simulink model "Trajectory_tracking_4th_order"  (R2024a)
settings: Solver=VariableStepAuto  StartTime=0.0  StopTime=tf  RelTol=1e-3
InitFcn:
  | %% Define the points of the curve
  | x=xp;
  | y=yp;
  | 
  | % Number of points
  | n = length(x);
  | 
  | % Initialize the arclength array
  | s = zeros(1, n);
  | 
  | %% Compute the incremental distances and the cumulative sum
  | for i = 2:n
  |     ds = sqrt((x(i) - x(i-1))^2 + (y(i) - y(i-1))^2);
  |     s(i) = s(i-1) + ds;
  | end
  | 
  | s= s/max(s);
  | 
  | [s, unique_indices] = unique(s, 'stable');
  | x = x(unique_indices);
  | y = y(unique_indices);
  | 
  | n = length(x);
  | 
  | %% Compute derivatives with respect to s
  | dx_ds = gradient(x, s);
  | dy_ds = gradient(y, s);
  | 
  | % Compute second derivatives with respect to s
  | d2x_ds2 = gradient(dx_ds, s);
  | d2y_ds2 = gradient(dy_ds, s);
  | 
  | % Compute third derivatives with respect to s
  | d3x_ds3 = gradient(d2x_ds2, s);
  | d3y_ds3 = gradient(d2y_ds2, s);
  | 
  | curvature = sqrt(d2x_ds2.^2+d2y_ds2.^2);
  | 
  | % % Dati Robot
  | %CGTF=0.325;
  | %CGTR=0.325;
  | Ts = 1/n;
  | 
  | 
  | %% Calcolo path
  | x_s= x;
  | y_s= y;
  | 
  | x_s_prime = dx_ds;
  | y_s_prime = dy_ds;
  | 
  | x_s_second = d2x_ds2;
  | y_s_second = d2y_ds2;
  | 
  | x_s_third = d3x_ds3;
  | y_s_third = d3y_ds3;
  | 
  | v_tilde = sqrt(x_s_prime.^2 + y_s_prime.^2);
  | 
  | theta_s = atan2(y_s_prime./v_tilde,x_s_prime./v_tilde);
  | theta_s_prime = (y_s_second.*x_s_prime-x_s_second.*y_s_prime)./(v_tilde.^2);
  | 
  | phi_s = atan(l*(y_s_second.*x_s_prime-x_s_second.*y_s_prime)./(v_tilde.^3));
  | 
  | w_tilde = (l*v_tilde.*((y_s_third.*x_s_prime-x_s_third.*y_s_prime)-3*(y_s_second.*x_s_prime-x_s_second.*y_s_prime).*(x_s_prime.*x_s_second+y_s_prime.*y_s_second)))./((v_tilde.^6)+(l^2)*(y_s_second.*x_s_prime-x_s_second.*y_s_prime).^2);
  | 
  | %% Time law
  | check=0;
  | t0 = 0;
  | %tf = 1;
  | K=1;
  | while (~check)
  | 
  |     a0 = s(:,1);
  |     a1 = 0;
  |     a2 = 3/(tf^2)*(s(:,n)-s(:,1));
  |     a3 = -2/(tf^3)*(s(:,n)-s(:,1));
  | 
  |     % % Define the boundary conditions for s(t)
  |     % t0 = 0; % initial time
  |     % t_end = tf; % end time
  |     % s0 = s(:,1); % initial arc length
  |     % s_end = s(:,n); % end arc length
  |     % v0 = 0; % initial velocity
  |     % v_end = 0; % end velocity
  |     % a0 = 0; % initial acceleration
  |     % a_end = 0; % end acceleration
  |     %
  |     % % Set up the system of equations for quintic polynomial
  |     % A = [
  |     %     1, t0, t0^2, t0^3, t0^4, t0^5;
  |     %     1, t_end, t_end^2, t_end^3, t_end^4, t_end^5;
  |     %     0, 1, 2*t0, 3*t0^2, 4*t0^3, 5*t0^4;
  |     %     0, 1, 2*t_end, 3*t_end^2, 4*t_end^3, 5*t_end^4;
  |     %     0, 0, 2, 6*t0, 12*t0^2, 20*t0^3;
  |     %     0, 0, 2, 6*t_end, 12*t_end^2, 20*t_end^3
  |     % ];
  |     %
  |     % b = [s0; s_end; v0; v_end; a0; a_end];
  |     %
  |     % % Solve for the coefficients
  |     % coefficients = A\b;
  |     %
  |     % % Extract the coefficients
  |     % a0 = coefficients(1);
  |     % a1 = coefficients(2);
  |     % a2 = coefficients(3);
  |     % a3 = coefficients(4);
  |     % a4 = coefficients(5);
  |     % a5 = coefficients(6);
  | 
  |     % Define the quintic polynomial function s(t)
  |     % s_t = @(t) a0 + a1*t + a2*t^2 + a3*t^3 + a4*t^4 + a5*t^5;
  |     s_t = @(t) a3*t^3 + a2*t^2 + a1*t + a0;
  | 
  |     % Create x(t) and y(t)
  |     x_t = @(t) interp1(s, x_s, s_t(t),'spline','extrap');
  |     y_t = @(t) interp1(s, y_s, s_t(t),'spline','extrap');
  | 
  |     t_values = linspace(0, tf, n);
  | 
  |     x_values = arrayfun(@(t) x_t(t),t_values);
  |     y_values = arrayfun(@(t) y_t(t),t_values);
  | 
  |     s_t_dot = 3*a3*t_values.^2 + 2*a2*t_values + a1;
  |     % s_t_dot = a1 + 2*a2*t_values + 3*a3*t_values.^2 + 4*a4*t_values.^3 + 5*a5*t_values.^4;
  | 
  |     x_t_dot = x_s_prime.*s_t_dot;
  |     y_t_dot = y_s_prime.*s_t_dot;
  | 
  |     v_t = v_tilde.*s_t_dot;
  | 
  |     w_t = w_tilde.*s_t_dot;
  | 
  |     theta_t = @(t) interp1(s, theta_s, s_t(t),'spline','extrap');
  |     theta_values = arrayfun(@(t) theta_t(t),t_values);
  | 
  |     theta_t_dot = theta_s_prime.*s_t_dot;
  | 
  |     phi_t = @(t) interp1(s, phi_s, s_t(t),'spline','extrap');
  |     phi_values = arrayfun(@(t) phi_t(t),t_values);
  | 
  |     theta_t_dot_lim = tan(phi_lim)/l*vlim;
  | 
  |     v_max = max(abs(v_t));
  |     w_max = max(abs(w_t));
  |     theta_max = max(abs(theta_t_dot));
  |     phi_max = max(abs(phi_values));
  | 
  |     check = 1;
  | 
  |     if ((v_max>vlim || w_max>wlim || theta_max>theta_t_dot_lim)) %&& phi_max<phi_lim )
  |         Kmax = [v_max/vlim w_max/wlim theta_max/theta_t_dot_lim ];
  |         K = max(Kmax);
  |         tf = tf*K;
  |         check=0;
  |     end
  | 
  | end
  | 
  | 
  | v_t_reference = timeseries(v_t,t_values);
  | w_t_reference = timeseries(w_t,t_values);
  | theta_t_reference = timeseries(theta_values,t_values);
  | theta_t_dot_reference = timeseries(theta_t_dot,t_values);
  | phi_t_reference = timeseries(phi_values,t_values);
  | 
  | x_t_reference = timeseries(x_values,t_values);
  | y_t_reference = timeseries(y_values,t_values);
  | x_dot_t_reference = timeseries(x_t_dot,t_values);
  | y_dot_t_reference = timeseries(y_t_dot,t_values);
values from neighbouring files (symbols this model uses):
  b = 5    [main.m]
  k1 = 30    [main.m]
  k2 = 3    [main.m]
undefined symbols (not defined in the file or in its folder): l, phi_lim, vlim, wlim
settings Model: Creator=arsen  LastModifiedBy=arsen

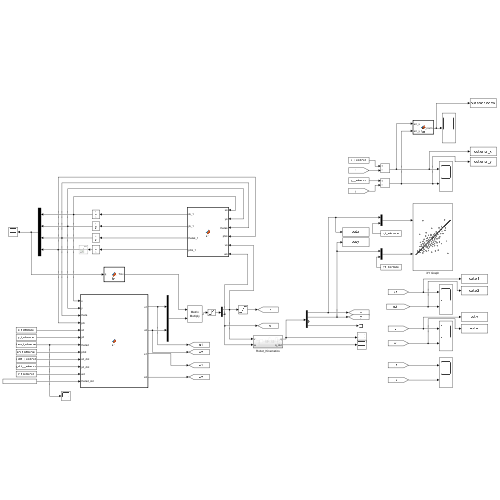
[thumbnail: Simulink's stored preview of the top-level diagram]
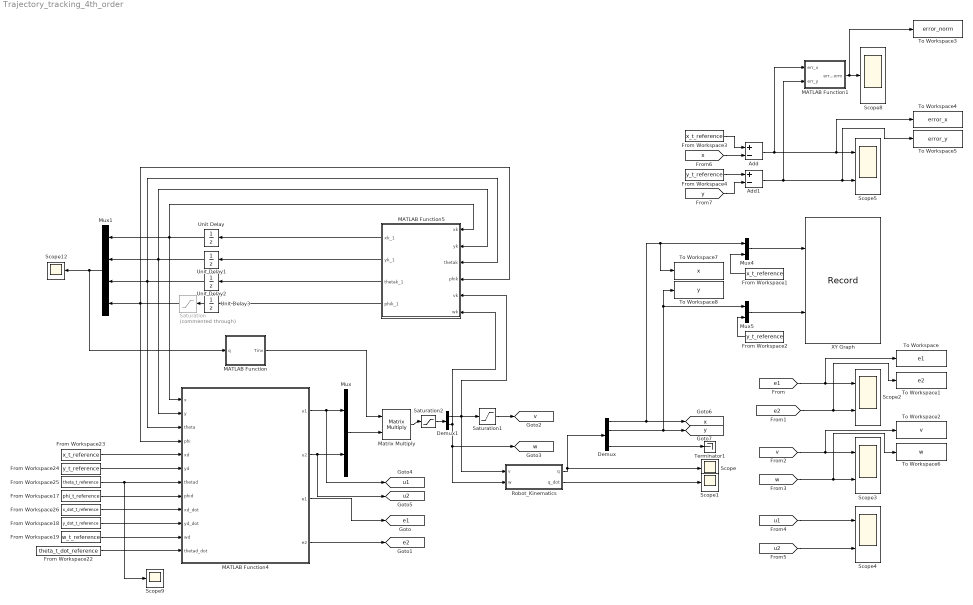
== system Trajectory_tracking_4th_order ==
  Add : Sum  Inputs=+-
  Add1 : Sum  Inputs=+-
  Demux : Demux
  Demux1 : Demux  Outputs=2
  From Workspace1 : FromWorkspace  VariableName=x_t_reference  SampleTime=Ts  OutputAfterFinalValue=Holding final value
  From Workspace17 : FromWorkspace  VariableName=phi_t_reference  OutDataTypeStr=double  SampleTime=Ts  OutputAfterFinalValue=Holding final value
  From Workspace18 : FromWorkspace  VariableName=y_dot_t_reference  OutDataTypeStr=double  SampleTime=Ts  OutputAfterFinalValue=Holding final value
  From Workspace19 : FromWorkspace  VariableName=w_t_reference  OutDataTypeStr=double  SampleTime=Ts  OutputAfterFinalValue=Holding final value
  From Workspace2 : FromWorkspace  VariableName=y_t_reference  SampleTime=Ts  OutputAfterFinalValue=Holding final value
  From Workspace22 : FromWorkspace  VariableName=theta_t_dot_reference  OutDataTypeStr=double  SampleTime=Ts  OutputAfterFinalValue=Holding final value
  From Workspace23 : FromWorkspace  VariableName=x_t_reference  OutDataTypeStr=double  SampleTime=Ts  OutputAfterFinalValue=Holding final value
  From Workspace24 : FromWorkspace  VariableName=y_t_reference  OutDataTypeStr=double  SampleTime=Ts  OutputAfterFinalValue=Holding final value
  From Workspace25 : FromWorkspace  VariableName=theta_t_reference  OutDataTypeStr=double  SampleTime=Ts  OutputAfterFinalValue=Holding final value
  From Workspace26 : FromWorkspace  VariableName=x_dot_t_reference  OutDataTypeStr=double  SampleTime=Ts  OutputAfterFinalValue=Holding final value
  From Workspace3 : FromWorkspace  VariableName=x_t_reference  SampleTime=Ts  OutputAfterFinalValue=Holding final value
  From Workspace4 : FromWorkspace  VariableName=y_t_reference  SampleTime=Ts  OutputAfterFinalValue=Holding final value
  MATLAB Function : MATLAB Function  TreatAsAtomicUnit=on
  MATLAB Function1 : MATLAB Function  TreatAsAtomicUnit=on
  MATLAB Function4 : MATLAB Function  TreatAsAtomicUnit=on
  MATLAB Function5 : MATLAB Function  TreatAsAtomicUnit=on
  Matrix Multiply : Product  Multiplication=Matrix(*)
  Mux : Mux  Inputs=2
  Mux1 : Mux
  Mux4 : Mux  Inputs=2
  Mux5 : Mux  Inputs=2
  Robot_Kinematics : Subsystem
  Saturation : Saturate  Commented=through  UpperLimit=phi_lim  LowerLimit=-phi_lim
  Saturation1 : Saturate  UpperLimit=inf  LowerLimit=0
  Saturation2 : Saturate  UpperLimit=[vlim wlim]'  LowerLimit=-[vlim wlim]'
  Scope{,1,8..9,12} (5 alike) : Scope
  Scope{2..5} (4 alike) : Scope  NumInputPorts=2
  Terminator1 : Terminator
  To Workspace : ToWorkspace  VariableName=e1  SaveFormat=Timeseries  SampleTime=-1
  To Workspace1 : ToWorkspace  VariableName=e2  SaveFormat=Timeseries  SampleTime=-1
  To Workspace2 : ToWorkspace  VariableName=v  SaveFormat=Timeseries  SampleTime=-1
  To Workspace3 : ToWorkspace  VariableName=error_norm  SaveFormat=Timeseries  SampleTime=-1
  To Workspace4 : ToWorkspace  VariableName=error_x  SaveFormat=Timeseries  SampleTime=-1
  To Workspace5 : ToWorkspace  VariableName=error_y  SaveFormat=Timeseries  SampleTime=-1
  To Workspace6 : ToWorkspace  VariableName=w  SaveFormat=Timeseries  SampleTime=-1
  To Workspace7 : ToWorkspace  VariableName=x  SaveFormat=Timeseries  SampleTime=-1
  To Workspace8 : ToWorkspace  VariableName=y  SaveFormat=Timeseries  SampleTime=-1
  Unit Delay : UnitDelay  InitialCondition=x_values(:,1)  SampleTime=Ts  HasFrameUpgradeWarning=on
  Unit Delay1 : UnitDelay  InitialCondition=y_values(:,1)  SampleTime=Ts  HasFrameUpgradeWarning=on
  Unit Delay2 : UnitDelay  InitialCondition=theta_values(:,1)  SampleTime=Ts  HasFrameUpgradeWarning=on
  Unit Delay3 : UnitDelay  InitialCondition=phi_values(:,1)  SampleTime=Ts  HasFrameUpgradeWarning=on
  XY Graph : Record  FileSettingsInternal="{\"entries\":[{\"content\":{\"excelSettings\":{\"content\":{},\"type\":\"Streamout.ExcelSettings\"}},\"type\":\"Streamout.FileSettingStorage\",\"uuid\":\"\"}],\"packageUris\":[\"http:\\/\\/schema.mathworks.com\\/mf0\\/streamout_blocks\\/R2020a\"],\"version\":\"1.0\"}"  Layout=[1 1]  SignalsInternal="{\"entries\":[{\"content\":{\"signals\":[{\"content\":{\"blockPath\":[],\"dimensions\":[2],\"domain\":\"\",\"hasChildren\":true,\"lineColor\":\"#ff13a6\",\"port\":1,\"signalID\":1,\"signalName\":\"Mux4\"},\"type\":\"RecordBlkView.Signal\",\"uuid\":\"\"},{\"content\":{\"blockPath\":[],\"channel\":[1],\"dimensions\":[2],\"domain\":\"\",\"lineColor\":\"#b746ff\",\"parentID\":1,\"plots\":[ 1 ],\"port\":1,\"signalID\":2,\"signalName\":\"Mux4\"},\"type\":\"RecordBlkView.Signal\",\"uuid\":\"\"},{\"content\":{\"blockPath\":[],\"channel\":[2],\"dimensions\":[2],\"domain\":\"\",\"lineColor\":\"#fe330a\",\"parentID\":1,\"plots\":[ 1 ],\"port\":1,\"signalID\":3,\"signalName\":\"Mux4\"},\"type\":\"RecordBlkView.Signal\",\"uuid\":\"\"},{\"content\":{\"blockPath\":[],\"dimensions\":[2],\"domain\":\"\",\"hasChildren\":true,\"lineColor\":\"#22b573\",\"port\":2,\"signalID\":4,\"signalName\":\"Mux5\"},\"type\":\"RecordBlkView.Signal\",\"uuid\":\"\"},{\"content\":{\"blockPath\":[],\"channel\":[1],\"dimensions\":[2],\"domain\":\"\",\"lineColor\":\"#ff13a6\",\"parentID\":4,\"plots\":[ 1 ],\"port\":2,\"signalID\":5,\"signalName\":\"Mux5\"},\"type\":\"RecordBlkView.Signal\",\"uuid\":\"\"},{\"content\":{\"blockPath\":[],\"channel\":[2],\"dimensions\":[2],\"domain\":\"\",\"lineColor\":\"#22b573\",\"parentID\":4,\"plots\":[ 1 ],\"port\":2,\"signalID\":6,\"signalName\":\"Mux5\"},\"type\":\"RecordBlkView.Signal\",\"uuid\":\"\"}]},\"type\":\"RecordBlkView.InputSignals\",\"uuid\":\"\"}],\"packageUris\":[\"http:\\/\\/schema.mathworks.com\\/mf0\\/streamout_blocks\\/R2020a\"],\"version\":\"1.0\"}"  VisualizationBindings="{\"xyplotplugin\":{\"info\":[{\"series\":[{\"bindingParametersList\":[{\"parameter\":\"X-Axis\",\"signalID\":2,\"signalName\":\"Mux4(1)\"},{\"parameter\":\"Y-Axis\",\"signalID\":5,\"signalName\":\"Mux5(1)\"}],\"seriesID\":0},{\"bindingParametersList\":[{\"parameter\":\"X-Axis\",\"signalID\":3,\"signalName\":\"Mux4(2)\"},{\"parameter\":\"Y-Axis\",\"signalID\":6,\"signalName\":\"Mux5(2)\"}],\"seriesID\":1}],\"subplotID\":1}]}}"  CompatibilityTag=XY
  tag scope: e1=global, e2=global, u1=global, u2=global, v=global, w=global, x=global, y=global
  wires:
  Mux4/1 -> XY Graph/1
  [e2] -> To Workspace1/1, Scope2/2
  [w] -> To Workspace6/1, Scope3/2
  From Workspace17/1 -> MATLAB Function4/8(phid)
  From Workspace18/1 -> MATLAB Function4/10(yd_dot)
  [v] -> To Workspace2/1, Scope3/1
  From Workspace1/1 -> Mux4/2
  MATLAB Function5/2(yk_1) -> Unit Delay1/1
  Add/1 -> MATLAB Function1/1(err_x), To Workspace4/1, Scope5/1
  Mux1/1 -> MATLAB Function/1(q), Scope12/1
  From Workspace23/1 -> MATLAB Function4/5(xd)
  MATLAB Function5/4(phik_1) -> Unit Delay3/1
  Mux5/1 -> XY Graph/2
  [u2] -> Scope4/2
  From Workspace2/1 -> Mux5/2
  From Workspace25/1 -> Scope9/1, MATLAB Function4/7(thetad)
  From Workspace22/1 -> MATLAB Function4/12(thetad_dot)
  From Workspace26/1 -> MATLAB Function4/9(xd_dot)
  From Workspace19/1 -> MATLAB Function4/11(wd)
  Saturation2/1 -> Demux1/1
  Saturation1/1 -> [v]
  [y] -> Add1/2
  MATLAB Function/1(Tinv) -> Matrix Multiply/1
  From Workspace4/1 -> Add1/1
  Demux/2 -> [y], To Workspace8/1, Mux5/1
  MATLAB Function4/1(u1) -> [u1], Mux/1
  Demux/4 -> Terminator1/1
  Matrix Multiply/1 -> Saturation2/1
  MATLAB Function1/1(err_norm) -> To Workspace3/1, Scope8/1
  [u1] -> Scope4/1
  Demux/1 -> To Workspace7/1, Mux4/1, [x]
  Demux1/1 -> Saturation1/1, Robot_Kinematics/1(v), MATLAB Function5/5(vk)
  Unit Delay3/1 -> Saturation/1
  From Workspace3/1 -> Add/1
  Unit Delay1/1 -> MATLAB Function5/2(yk), Mux1/2, MATLAB Function4/2(y)
  MATLAB Function4/3(e1) -> [e1]
  Unit Delay2/1 -> MATLAB Function4/3(theta), MATLAB Function5/3(thetak), Mux1/3
  MATLAB Function4/2(u2) -> [u2], Mux/2
  MATLAB Function5/3(thetak_1) -> Unit Delay2/1
  [e1] -> To Workspace/1, Scope2/1
  Mux/1 -> Matrix Multiply/2
  MATLAB Function4/4(e2) -> [e2]
  Saturation/1 -> MATLAB Function4/4(phi), MATLAB Function5/4(phik), Mux1/4
  Robot_Kinematics/1(q) -> Scope/1, Demux/1
  Unit Delay/1 -> MATLAB Function5/1(xk), Mux1/1, MATLAB Function4/1(x)
  Demux1/2 -> [w], Robot_Kinematics/2(w), MATLAB Function5/6(wk)
  Add1/1 -> MATLAB Function1/2(err_y), To Workspace5/1, Scope5/2
  MATLAB Function5/1(xk_1) -> Unit Delay/1
  From Workspace24/1 -> MATLAB Function4/6(yd)
  Robot_Kinematics/2(q_dot) -> Scope1/1
  [x] -> Add/2

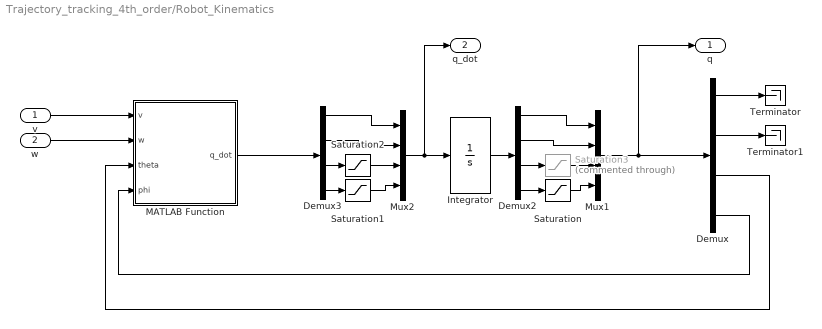
== system Trajectory_tracking_4th_order/Robot_Kinematics ==
  v : Inport
  w : Inport  Port=2
  Demux : Demux
  Demux2 : Demux
  Demux3 : Demux
  Integrator : Integrator  InitialCondition=[x_values(:,1) y_values(:,1) theta_values(:,1) phi_values(:,1)]'  UpperSaturationLimit=[inf inf inf 1.5]'  LowerSaturationLimit=[-inf -inf -inf -1.5]'
  MATLAB Function : MATLAB Function  TreatAsAtomicUnit=on
  Mux1 : Mux
  Mux2 : Mux
  Saturation : Saturate  UpperLimit=phi_lim  LowerLimit=-phi_lim
  Saturation1 : Saturate  UpperLimit=wlim  LowerLimit=-wlim
  Saturation2 : Saturate  UpperLimit=theta_t_dot_lim  LowerLimit=-theta_t_dot_lim
  Saturation3 : Saturate  Commented=through  UpperLimit=2*pi  LowerLimit=-2*pi
  Terminator : Terminator
  Terminator1 : Terminator
  q : Outport
  q_dot : Outport  Port=2
  wires:
  Integrator/1 -> Demux2/1
  Demux/3 -> MATLAB Function/3(theta)
  Demux/4 -> MATLAB Function/4(phi)
  v/1 -> MATLAB Function/1(v)
  w/1 -> MATLAB Function/2(w)
  Demux/1 -> Terminator/1
  Demux/2 -> Terminator1/1
  Demux2/4 -> Saturation/1
  Mux1/1 -> q/1, Demux/1
  Saturation/1 -> Mux1/4
  Demux2/3 -> Saturation3/1
  Demux2/2 -> Mux1/2
  Demux2/1 -> Mux1/1
  Saturation1/1 -> Mux2/4
  Demux3/2 -> Mux2/2
  Demux3/4 -> Saturation1/1
  Demux3/3 -> Saturation2/1
  MATLAB Function/1(q_dot) -> Demux3/1
  Demux3/1 -> Mux2/1
  Mux2/1 -> q_dot/1, Integrator/1
  Saturation2/1 -> Mux2/3
  Saturation3/1 -> Mux1/3

== matlab function Trajectory_tracking_4th_order/MATLAB Function ==
  data: q input; Tinv output; b parameter; l parameter
function Tinv = fcn(q,b,l)

T = [cos(q(3))-tan(q(4))*sin(q(3))-(b/l)*tan(q(4))*sin(q(3)+q(4)) -b*sin(q(3)+q(4));
    sin(q(3))+tan(q(4))*cos(q(3))+(b/l)*tan(q(4))*cos(q(3)+q(4)) b*cos(q(3)+q(4))];


Tinv= inv(T);

== matlab function Trajectory_tracking_4th_order/Robot_Kinematics/MATLAB Function ==
  data: v input; q_dot output; w input; theta input; phi input; l parameter
function q_dot = fcn(v,w,theta,phi,l)

x_dot = cos(theta)*v;
y_dot = sin(theta)*v;
theta_dot = (tan(phi)/l)*v;
phi_dot = w;

q_dot = [x_dot y_dot theta_dot phi_dot]';

== matlab function Trajectory_tracking_4th_order/MATLAB Function1 ==
  data: err_x input; err_norm output; err_y input
function err_norm = fcn(err_x,err_y)


err_norm = sqrt((err_x^2)+(err_y^2));

== matlab function Trajectory_tracking_4th_order/MATLAB Function4 ==
  data: x input; u1 output; u2 output; y input; theta input; phi input; xd input; yd input; thetad input; phid input; xd_dot input; yd_dot input; wd input; thetad_dot input; e1 output; e2 output; b parameter; l parameter; Ts parameter; d2x_ds2 parameter; d2y_ds2 parameter; k1 parameter; k2 parameter
function [u1,u2,e1,e2]=fcn(x,y,theta,phi,xd,yd,thetad,phid,xd_dot,yd_dot,wd,thetad_dot,b,l,Ts,d2x_ds2, d2y_ds2,k1, k2)
% 
% persistent sum1;
% persistent sum2;

  
% 
% if isempty(sum1) || isempty(sum2) 
%          sum1 = 0;
%          sum2 = 0;
% end


e1 = (xd+l*cos(thetad)+b*cos(thetad+phid))-(x+l*cos(theta)+b*cos(theta+phi));
e2 = (yd+l*sin(thetad)+b*sin(thetad+phid))-(y+l*sin(theta)+b*sin(theta+phi));

% sum1=sum1+e1*Ts;
% sum2=sum2+e2*Ts;




% k1=3.5;
% k2=k1*(max(d2y_ds2)/max(d2x_ds2));
% k3=0;
% k4=0;

u1 = xd_dot-l*thetad_dot*sin(thetad)-b*(thetad_dot+wd)*sin(thetad+phid) + k1*e1; 
u2 = yd_dot+l*thetad_dot*cos(thetad)+b*(thetad_dot+wd)*cos(thetad+phid) + k2*e2;

== matlab function Trajectory_tracking_4th_order/MATLAB Function5 ==
  data: xk input; xk_1 output; yk input; thetak input; phik input; vk input; wk input; yk_1 output; thetak_1 output; Ts parameter; phik_1 output; l parameter
function [xk_1, yk_1 ,thetak_1,phik_1] = fcn(xk,yk,thetak,phik,vk,wk, Ts,l)

% xk_1 = xk + Ts*vk*cos(thetak+(0.5*Ts*vk/l*tan(phik)));
% yk_1 = yk + Ts*vk*sin(thetak+(0.5*Ts*vk/l*tan(phik)));
% thetak_1 = thetak + Ts*(vk/l*tan(phik));

% First step
k1_x = vk * cos(thetak);
k1_y = vk * sin(thetak);
k1_theta = vk / l * tan(phik);
phik_1 = phik + wk*Ts;

% Second step
k2_x = vk * cos(thetak + Ts / 2 * k1_theta);
k2_y = vk * sin(thetak + Ts / 2 * k1_theta);
k2_theta = vk / l * tan(phik);

% Third step
k3_x = vk * cos(thetak + Ts / 2 * k2_theta);
k3_y = vk * sin(thetak + Ts / 2 * k2_theta);
k3_theta = vk / l * tan(phik);

% Fourth step
k4_x = vk * cos(thetak + Ts * k3_theta);
k4_y = vk * sin(thetak + Ts * k3_theta);
k4_theta = vk / l * tan(phik);

% Update state
xk_1 = xk + Ts / 6 * (k1_x + 2 * k2_x + 2 * k3_x + k4_x);
yk_1 = yk + Ts / 6 * (k1_y + 2 * k2_y + 2 * k3_y + k4_y);
thetak_1 = thetak + Ts / 6 * (k1_theta + 2 * k2_theta + 2 * k3_theta + k4_theta);
